simulink model "chap2_12sim"  (Simulink 6.3)
settings: Solver=ode45  StartTime=0.0  StopTime=100  RelTol=1e-3
values from neighbouring files (symbols this model uses):
  a1 = 3    [chap2_12int.m]    (also in chap2_12save.mat)
  a2 = 43    [chap2_12int.m]    (also in chap2_12save.mat)
  kd = 10    [chap2_12int.m]    (also in chap2_12save.mat = 9.99804334002; chap2_4tuning.m = kp*pi/(4*wm); chap2_5tuning.m = kp*pi/(4*wm); chap2_8ctrl.m = -19)
  ki = 0.10    (= 0.1)    [chap2_12int.m]    (also in chap2_12save.mat = 0.0698139131399; chap2_4tuning.m = kp*wm/pi; chap2_5tuning.m = kp*wm/pi)
  kp = 1    [chap2_12int.m]    (also in chap2_12save.mat = 1.01140093599; chap2_4tuning.m = 0.6*km; chap2_5tuning.m = 0.6*km; chap2_8ctrl.m = 9)
libraries: simulink_extras x1
settings Model: LastModifiedBy=Administrator  ExtModeTrigMode=oneshot  ExtModeArmWhenConnect=off  StrictBusMsg=None
settings DataIOCC: LimitDataPoints=off  SignalLoggingName=sigsOut
settings OptimizationCC: BooleanDataType=off
settings DebuggingCC: SolverPrmCheckMsg=none
settings HardwareCC: TargetUnknown=on

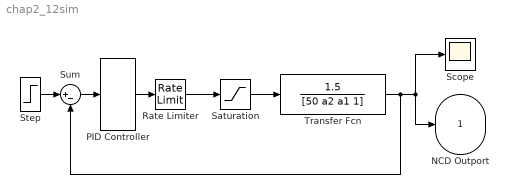
== system chap2_12sim ==
  PID Controller : simulink_extras/Additional Linear/PID Controller  P=kp  I=ki  D=kd
  Rate Limiter : RateLimiter  RisingSlewLimit=0.8  FallingSlewLimit=-0.8
  Saturation : Saturate  UpperLimit=1  LowerLimit=-1
  Scope : Scope
  Step : Step  SampleTime=0
  Sum : Sum  Inputs=|+-  SaturateOnIntegerOverflow=on  InputSameDT=on
  Transfer Fcn : TransferFcn  Numerator=[1.5]  Denominator=[50 a2 a1 1]
  NCD Outport : Outport  InitialOutput=0
      settings: OpenFcn=optblock
      mask Type: NCD Outport
      mask Display:
      | plot([0:10],[-.5 1.5 .6 1.3 .8 1.1 .95 1.02 .99 1 1]);
      | disp('\n\n NCD\n OutPort 1');
  wires:
  Sum/1 -> PID Controller/1
  Step/1 -> Sum/1
  PID Controller/1 -> Rate Limiter/1
  Rate Limiter/1 -> Saturation/1
  Saturation/1 -> Transfer Fcn/1
  Transfer Fcn/1 -> NCD Outport/1, Scope/1, Sum/2
